simulink model "lisan1"  (R2018b)
settings: Solver=VariableStepAuto  StartTime=0.0  StopTime=10.0  FixedStep=0.02  RelTol=1e-3
libraries: discretizing x3
settings Model: Creator=QJ-  LastModifiedBy=QJ-

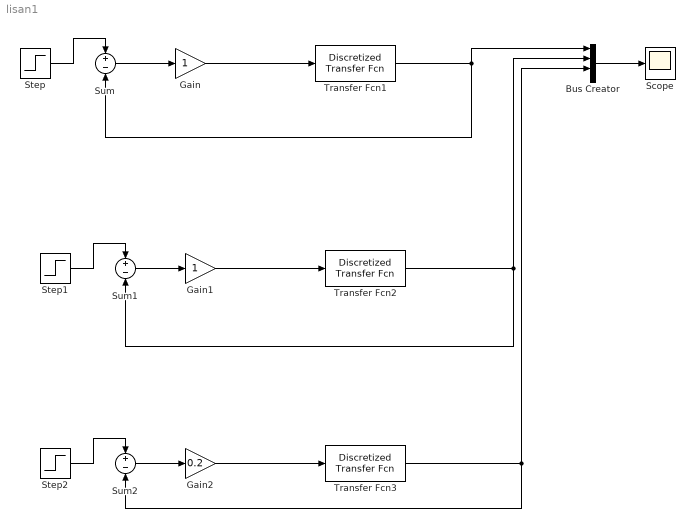
== system lisan1 ==
  Bus Creator : BusCreator  Inputs=4
  Gain : Gain
  Gain1 : Gain
  Gain2 : Gain  Gain=0.2
  Scope : Scope
  Step : Step  SampleTime=0.02
  Step1 : Step  SampleTime=0.05
  Step2 : Step  SampleTime=0.1
  Sum : Sum  Inputs=+-
  Sum1 : Sum  Inputs=+-
  Sum2 : Sum  Inputs=+-
  Transfer Fcn1 : discretizing/Discretized Transfer Fcn  Numerator=[20]  Denominator=[0.1 1 0]  AbsTol=auto  SampleTime=0.02  method=zoh  Wc=0
  Transfer Fcn2 : discretizing/Discretized Transfer Fcn  Numerator=[20]  Denominator=[0.1 1 0]  AbsTol=auto  SampleTime=0.05  method=zoh  Wc=0
  Transfer Fcn3 : discretizing/Discretized Transfer Fcn  Numerator=[20]  Denominator=[0.1 1 0]  AbsTol=auto  SampleTime=0.1  method=zoh  Wc=0
  wires:
  Step/1 -> Sum/1
  Sum/1 -> Gain/1
  Bus Creator/1 -> Scope/1
  Gain/1 -> Transfer Fcn1/1
  Transfer Fcn1/1 -> Bus Creator/1, Sum/2
  Gain1/1 -> Transfer Fcn2/1
  Sum1/1 -> Gain1/1
  Transfer Fcn2/1 -> Bus Creator/2, Sum1/2
  Step1/1 -> Sum1/1
  Gain2/1 -> Transfer Fcn3/1
  Sum2/1 -> Gain2/1
  Step2/1 -> Sum2/1
  Transfer Fcn3/1 -> Bus Creator/3, Sum2/2
